simulink model "CoTS_ThermDem"  (R2016b)
settings: configuration reference "CodeGenConfigSet" (kept outside this file)
values from neighbouring files (symbols this model uses):
  CoTS_facPT1Neg_C = Calibration.Parameter    [init_CoTS_ThermDem.m]
  CoTS_facPT1Pos_C = Calibration.Parameter    [init_CoTS_ThermDem.m]
  CoTS_tClntEngOutDes_C = Calibration.Parameter    [init_CoTS_ThermDem.m]
libraries: CXLib x1
settings Model: Creator=xinchangran  LastModifiedBy=xinchangran
settings ConfigSetRef: SourceLocation=Base Workspace

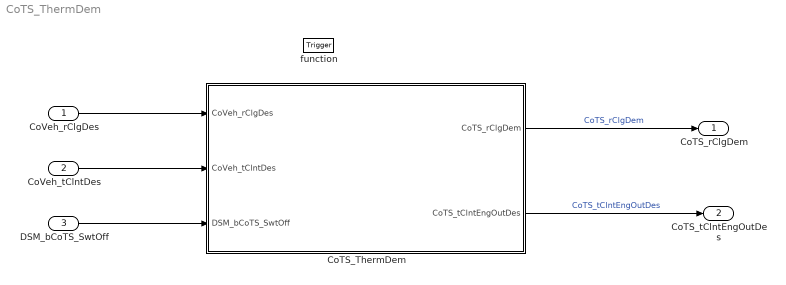
== system CoTS_ThermDem ==
  CoVeh_rClgDes : Inport  Tag=%  Description=Desired relative air mass flow  OutMin=-300  OutMax=300  OutDataTypeStr=Prc_100_rate
  CoVeh_tClntDes : Inport  Tag=deg  Description=Desired coolant temperature  Port=2  OutMin=-150  OutMax=150  OutDataTypeStr=Temp_deg
  DSM_bCoTS_SwtOff : Inport  Description=Use of replacement value for desired engine coolant temperature  Port=3  OutMin=0  OutMax=1  OutDataTypeStr=boolean
  function : TriggerPort  TriggerType=function-call  VariantControl=Variant
  CoTS_ThermDem : Subsystem
  CoTS_rClgDem : Outport  Tag=%  Description=cool demand percent  OutMin=-300  OutMax=300  OutDataTypeStr=Prc_100_rate
  CoTS_tClntEngOutDes : Outport  Tag=deg  Description=Coolant temperature of combustion engine  Port=2  OutMin=-3549  OutMax=3003  OutDataTypeStr=Temp_deg
  wires:
  CoVeh_rClgDes/1 -> CoTS_ThermDem/1(CoVeh_rClgDes)
  CoVeh_tClntDes/1 -> CoTS_ThermDem/2(CoVeh_tClntDes)
  DSM_bCoTS_SwtOff/1 -> CoTS_ThermDem/3(DSM_bCoTS_SwtOff)
  CoTS_ThermDem/1(CoTS_rClgDem) -> CoTS_rClgDem/1  "CoTS_rClgDem"
  CoTS_ThermDem/2(CoTS_tClntEngOutDes) -> CoTS_tClntEngOutDes/1  "CoTS_tClntEngOutDes"

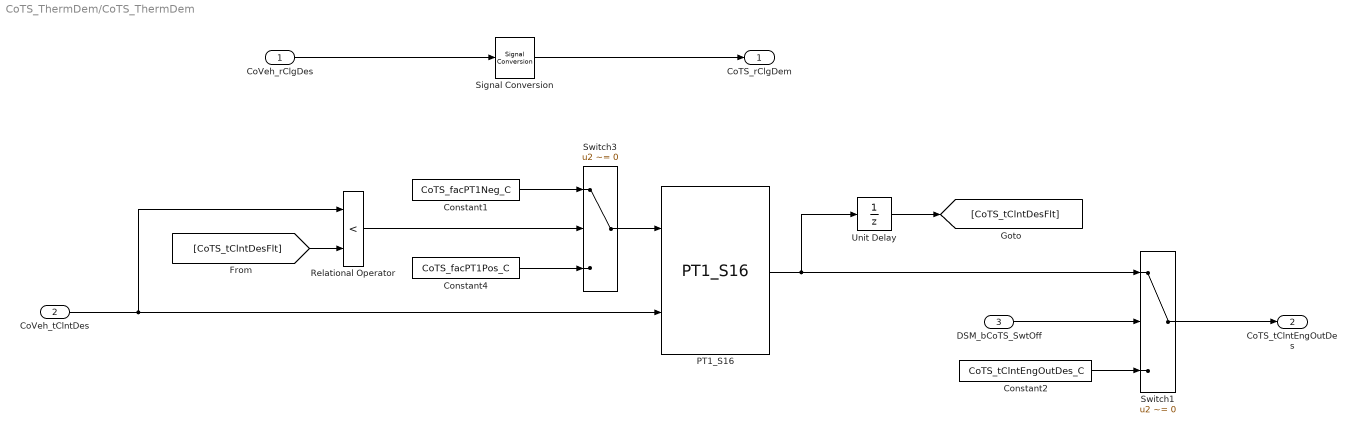
== system CoTS_ThermDem/CoTS_ThermDem ==
  CoVeh_rClgDes : Inport  Tag=%  Description=Desired relative air mass flow
  CoVeh_tClntDes : Inport  Tag=deg  Description=Desired coolant temperature  Port=2
  DSM_bCoTS_SwtOff : Inport  Description=Use of replacement value for desired engine coolant temperature  Port=3  OutMin=0  OutMax=1  OutDataTypeStr=boolean
  Constant1 : Constant  Value=CoTS_facPT1Neg_C
  Constant2 : Constant  Value=CoTS_tClntEngOutDes_C
  Constant4 : Constant  Value=CoTS_facPT1Pos_C
  PT1_S16 : CXLib/PT1_S16
  Relational Operator : RelationalOperator  Operator=<  OutDataTypeStr=boolean  RndMeth=Simplest
  Signal Conversion : SignalConversion  OverrideOpt=off
  Switch1 : Switch  Criteria=u2 ~= 0  SaturateOnIntegerOverflow=on  InputSameDT=on
  Switch3 : Switch  Criteria=u2 ~= 0  SaturateOnIntegerOverflow=on  InputSameDT=on
  Unit Delay : UnitDelay  SampleTime=-1
      settings: AttributesFormatString=InitialValue=%<InitialCondition>
  CoTS_rClgDem : Outport  Tag=%  Description=cool demand percent
  CoTS_tClntEngOutDes : Outport  Tag=deg  Description=Coolant temperature of combustion engine  Port=2
  wires:
  Switch1/1 -> CoTS_tClntEngOutDes/1
  Signal Conversion/1 -> CoTS_rClgDem/1
  DSM_bCoTS_SwtOff/1 -> Switch1/2
  Constant2/1 -> Switch1/3
  CoVeh_tClntDes/1 -> Relational Operator/1, PT1_S16/2
  Switch3/1 -> PT1_S16/1
  Constant1/1 -> Switch3/1
  Relational Operator/1 -> Switch3/2
  Constant4/1 -> Switch3/3
  PT1_S16/1 -> Unit Delay/1, Switch1/1
  [CoTS_tClntDesFlt] -> Relational Operator/2
  CoVeh_rClgDes/1 -> Signal Conversion/1
  Unit Delay/1 -> [CoTS_tClntDesFlt]
